simulink subsystem "visualization_nav"  (R2026a)
settings: Solver=VariableStepAuto
undefined symbols (not defined in the file): location
libraries: aerolibanim x1, dspindex x1, sharedtransform x1
settings Model: Creator=finnb  LastModifiedBy=trist

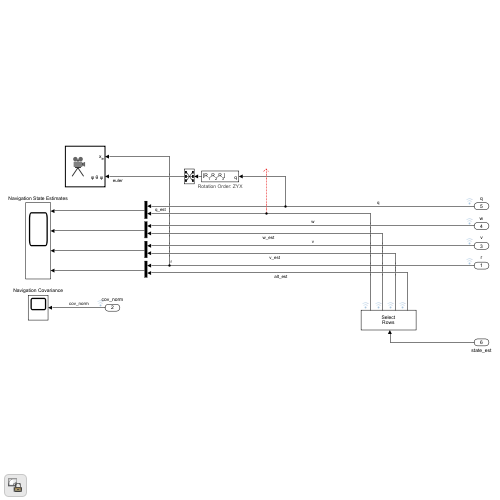
[thumbnail: Simulink's stored preview of the top-level diagram]
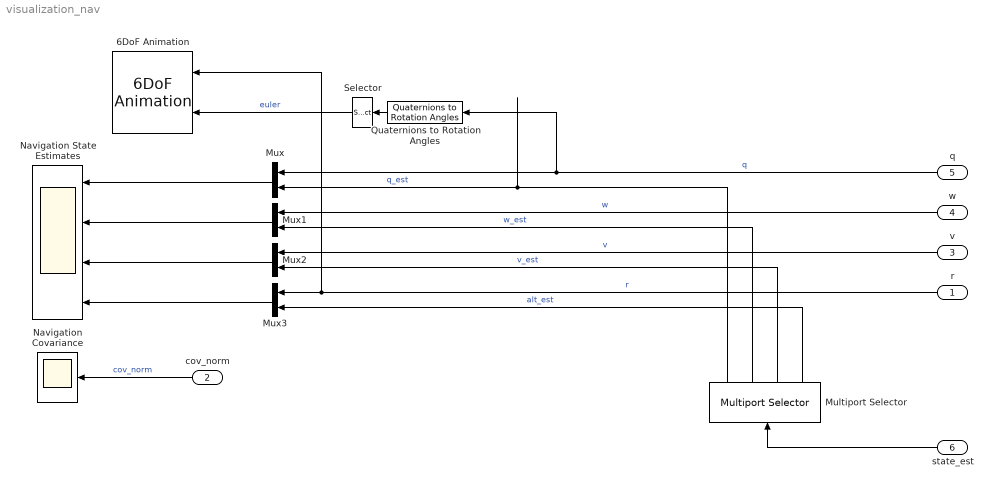
== system visualization_nav ==
  r : Inport
  cov_norm : Inport  Port=2
  v : Inport  Port=3
  w : Inport  Port=4
  q : Inport  Port=5
  state_est : Inport  Port=6
  6DoF Animation : aerolibanim/6DoF Animation  u1=[0 8000 -100 100 0 400]  u2=0.1  u3=5  u4=[location(1)-5 0 0]  u5=Fly alongside  u6=[0 100 0]  u7=10  u8=off
  Multiport Selector : dspindex/Multiport Selector  rowsOrCols=Rows  idxCellArray={ 1:4, 5:7, 8:10, 11}  idxErrMode=Clip Index
  Mux : Mux  Inputs=[4 4]
  Mux1 : Mux  Inputs=2
  Mux2 : Mux  Inputs=2
  Mux3 : Mux  Inputs=2
  Navigation Covariance : Scope
      settings: Title=Covariance Nrom  ActiveDisplayYMinimum=-3.2752028005364187  ActiveDisplayYMaximum=29.476825204827776  DataLoggingVariableName=ScopeData2
  Navigation State Estimates : Scope  NumInputPorts=4
      settings: Title=Attitude Quaternion  ActiveDisplayYMinimum=-1.2396783312686264  ActiveDisplayYMaximum=1.2473304087571517  DataLoggingVariableName=ScopeData11
  Quaternions to Rotation Angles : sharedtransform/Quaternions to Rotation Angles  rotationOrder=ZYX  aMode=aMode
  Selector : Selector  InputPortWidth=3  IndexOptions=Index vector (dialog)  Indices=[3 2 1]  OutputSizes=1
  wires:
  q/1 -> Mux/1, Quaternions to Rotation Angles/1  "q"
  w/1 -> Mux1/1  "w"
  Mux2/1 -> Navigation State Estimates/3
  Multiport Selector/1 -> Mux/2  "q_est"
  state_est/1 -> Multiport Selector/1
  Multiport Selector/4 -> Mux3/2  "alt_est"
  Selector/1 -> 6DoF Animation/2  "euler"
  Mux1/1 -> Navigation State Estimates/2
  Multiport Selector/2 -> Mux1/2  "w_est"
  Multiport Selector/3 -> Mux2/2  "v_est"
  Mux/1 -> Navigation State Estimates/1
  Mux3/1 -> Navigation State Estimates/4
  v/1 -> Mux2/1  "v"
  r/1 -> 6DoF Animation/1, Mux3/1  "r"
  Quaternions to Rotation Angles/1 -> Selector/1
  cov_norm/1 -> Navigation Covariance/1  "cov_norm"
